simulink model "FOC_HF_G474"  (R2020b)
settings: Solver=FixedStepDiscrete  StartTime=0.0  StopTime=10  FixedStep=TsBSP  RelTol=1e-3
values from neighbouring files (symbols this model uses):
  BandwidthCurrentPI = 314.15926535897933    [G474_FOC_HF.sldd]
  Ld = 4.9E-5    [G474_FOC_HF.sldd]    (also in Hall_HFI_FOC_Data.sldd = 0.0004
  Ld_MODEL = 4.9E-5    [G474_FOC_HF.sldd]
  Lq = 4.9E-5    [G474_FOC_HF.sldd]    (also in Hall_HFI_FOC_Data.sldd = 0.00045
  Lq_MODEL = 4.9E-5    [G474_FOC_HF.sldd]
  MaxVoltage = 5.0    [G474_FOC_HF.sldd]
  PolePairs = 5.0    [G474_FOC_HF.sldd]
  PolePairs_MODEL = 5.0    [G474_FOC_HF.sldd]
  PWMHalfPeriod = 4199.0    [G474_FOC_HF.sldd]
  Rs = 0.082    [G474_FOC_HF.sldd]
  TsBSP = 2.0E-5    [G474_FOC_HF.sldd]
  TsFOC = 0.0001    [G474_FOC_HF.sldd]
  TsFOC_MODEL = 0.0001    [G474_FOC_HF.sldd]
undefined symbols (not defined in the file or in its folder): sigbuilder_block
libraries: pid_lib x4, mcbplantlib x1, autolibpmsminterior x1
(part 2 of 2)

== system FOC_HF_G474/FOC/FOC_CURRENT/SVPWM/CalcPWM/Switch Case Action Subsystem/tLimit ==
  t1 : Inport
  t2 : Inport  Port=2
  PWMHalfPeriod : Inport  Port=3
  If : If  IfExpression=u1
  If Action Subsystem : Subsystem  TreatAsAtomicUnit=on
  If Action Subsystem1 : Subsystem  TreatAsAtomicUnit=on
  Merge : Merge
  Merge1 : Merge
  Relational Operator : RelationalOperator  Operator=>  OutDataTypeStr=boolean  RndMeth=Simplest
  Sum4 : Sum  Inputs=|++
  t1Limit : Outport
  t2Limit : Outport  Port=2
  wires:
  t2/1 -> If Action Subsystem1/2(t2), If Action Subsystem/2(t2), Sum4/2
  Sum4/1 -> Relational Operator/1
  If/1 -> If Action Subsystem/Action
  Relational Operator/1 -> If/1
  PWMHalfPeriod/1 -> Relational Operator/2, If Action Subsystem/3(PWMHalfPeriod)
  t1/1 -> If Action Subsystem1/1(t1), If Action Subsystem/1(t1), Sum4/1
  If/2 -> If Action Subsystem1/Action
  If Action Subsystem/1(t1Limit) -> Merge/1
  If Action Subsystem1/1(t1Limit) -> Merge/2
  Merge/1 -> t1Limit/1
  If Action Subsystem1/2(t2Limit) -> Merge1/2
  If Action Subsystem/2(t2Limit) -> Merge1/1
  Merge1/1 -> t2Limit/1

== system FOC_HF_G474/FOC/FOC_CURRENT/SVPWM/CalcPWM/Switch Case Action Subsystem1/tLimit ==
  t2 : Inport
  t3 : Inport  Port=2
  PWMHalfPeriod : Inport  Port=3
  If : If  IfExpression=u1
  If Action Subsystem : Subsystem  TreatAsAtomicUnit=on
  If Action Subsystem1 : Subsystem  TreatAsAtomicUnit=on
  Merge : Merge
  Merge1 : Merge
  Relational Operator : RelationalOperator  Operator=>  OutDataTypeStr=boolean  RndMeth=Simplest
  Sum4 : Sum  Inputs=|++
  t2Limit : Outport
  t3Limit : Outport  Port=2
  wires:
  t3/1 -> If Action Subsystem1/2(t3), If Action Subsystem/2(t3), Sum4/2
  Sum4/1 -> Relational Operator/1
  If/1 -> If Action Subsystem/Action
  Relational Operator/1 -> If/1
  PWMHalfPeriod/1 -> Relational Operator/2, If Action Subsystem/3(PWMHalfPeriod)
  t2/1 -> If Action Subsystem1/1(t2), If Action Subsystem/1(t2), Sum4/1
  If/2 -> If Action Subsystem1/Action
  If Action Subsystem/1(t2Limit) -> Merge/1
  If Action Subsystem1/1(t2Limit) -> Merge/2
  Merge/1 -> t2Limit/1
  If Action Subsystem1/2(t3Limit) -> Merge1/2
  If Action Subsystem/2(t3Limit) -> Merge1/1
  Merge1/1 -> t3Limit/1

== system FOC_HF_G474/FOC/FOC_CURRENT/SVPWM/CalcPWM/Switch Case Action Subsystem2/tLimit ==
  t4 : Inport
  t3 : Inport  Port=2
  PWMHalfPeriod : Inport  Port=3
  If : If  IfExpression=u1
  If Action Subsystem : Subsystem  TreatAsAtomicUnit=on
  If Action Subsystem1 : Subsystem  TreatAsAtomicUnit=on
  Merge : Merge
  Merge1 : Merge
  Relational Operator : RelationalOperator  Operator=>  OutDataTypeStr=boolean  RndMeth=Simplest
  Sum4 : Sum  Inputs=|++
  t4Limit : Outport
  t3Limit : Outport  Port=2
  wires:
  t3/1 -> If Action Subsystem1/2(t3), If Action Subsystem/2(t3), Sum4/2
  Sum4/1 -> Relational Operator/1
  If/1 -> If Action Subsystem/Action
  Relational Operator/1 -> If/1
  PWMHalfPeriod/1 -> Relational Operator/2, If Action Subsystem/3(PWMHalfPeriod)
  t4/1 -> If Action Subsystem1/1(t4), If Action Subsystem/1(t4), Sum4/1
  If/2 -> If Action Subsystem1/Action
  If Action Subsystem/1(t4Limit) -> Merge/1
  If Action Subsystem1/1(t4Limit) -> Merge/2
  Merge/1 -> t4Limit/1
  If Action Subsystem1/2(t3Limit) -> Merge1/2
  If Action Subsystem/2(t3Limit) -> Merge1/1
  Merge1/1 -> t3Limit/1

== system FOC_HF_G474/FOC/FOC_CURRENT/SVPWM/CalcPWM/Switch Case Action Subsystem3/tLimit ==
  t4 : Inport
  t5 : Inport  Port=2
  PWMHalfPeriod : Inport  Port=3
  If : If  IfExpression=u1
  If Action Subsystem : Subsystem  TreatAsAtomicUnit=on
  If Action Subsystem1 : Subsystem  TreatAsAtomicUnit=on
  Merge : Merge
  Merge1 : Merge
  Relational Operator : RelationalOperator  Operator=>  OutDataTypeStr=boolean  RndMeth=Simplest
  Sum4 : Sum  Inputs=|++
  t4Limit : Outport
  t5Limit : Outport  Port=2
  wires:
  t5/1 -> If Action Subsystem1/2(t5), If Action Subsystem/2(t5), Sum4/2
  Sum4/1 -> Relational Operator/1
  If/1 -> If Action Subsystem/Action
  Relational Operator/1 -> If/1
  PWMHalfPeriod/1 -> Relational Operator/2, If Action Subsystem/3(PWMHalfPeriod)
  t4/1 -> If Action Subsystem1/1(t4), If Action Subsystem/1(t4), Sum4/1
  If/2 -> If Action Subsystem1/Action
  If Action Subsystem/1(t4Limit) -> Merge/1
  If Action Subsystem1/1(t4Limit) -> Merge/2
  Merge/1 -> t4Limit/1
  If Action Subsystem1/2(t5Limit) -> Merge1/2
  If Action Subsystem/2(t5Limit) -> Merge1/1
  Merge1/1 -> t5Limit/1

== system FOC_HF_G474/FOC/FOC_CURRENT/SVPWM/CalcPWM/Switch Case Action Subsystem4/tLimit ==
  t5 : Inport
  t6 : Inport  Port=2
  PWMHalfPeriod : Inport  Port=3
  If : If  IfExpression=u1
  If Action Subsystem : Subsystem  TreatAsAtomicUnit=on
  If Action Subsystem1 : Subsystem  TreatAsAtomicUnit=on
  Merge : Merge
  Merge1 : Merge
  Relational Operator : RelationalOperator  Operator=>  OutDataTypeStr=boolean  RndMeth=Simplest
  Sum4 : Sum  Inputs=|++
  t5Limit : Outport
  t6Limit : Outport  Port=2
  wires:
  t6/1 -> If Action Subsystem1/2(t6), If Action Subsystem/2(t6), Sum4/2
  Sum4/1 -> Relational Operator/1
  If/1 -> If Action Subsystem/Action
  Relational Operator/1 -> If/1
  PWMHalfPeriod/1 -> Relational Operator/2, If Action Subsystem/3(PWMHalfPeriod)
  t5/1 -> If Action Subsystem1/1(t5), If Action Subsystem/1(t5), Sum4/1
  If/2 -> If Action Subsystem1/Action
  If Action Subsystem/1(t5Limit) -> Merge/1
  If Action Subsystem1/1(t5Limit) -> Merge/2
  Merge/1 -> t5Limit/1
  If Action Subsystem1/2(t6Limit) -> Merge1/2
  If Action Subsystem/2(t6Limit) -> Merge1/1
  Merge1/1 -> t6Limit/1

== system FOC_HF_G474/FOC/FOC_CURRENT/SVPWM/CalcPWM/Switch Case Action Subsystem5/tLimit ==
  t1 : Inport
  t6 : Inport  Port=2
  PWMHalfPeriod : Inport  Port=3
  If : If  IfExpression=u1
  If Action Subsystem : Subsystem  TreatAsAtomicUnit=on
  If Action Subsystem1 : Subsystem  TreatAsAtomicUnit=on
  Merge : Merge
  Merge1 : Merge
  Relational Operator : RelationalOperator  Operator=>  OutDataTypeStr=boolean  RndMeth=Simplest
  Sum4 : Sum  Inputs=|++
  t1Limit : Outport
  t6Limit : Outport  Port=2
  wires:
  t6/1 -> If Action Subsystem1/2(t6), If Action Subsystem/2(t6), Sum4/2
  Sum4/1 -> Relational Operator/1
  If/1 -> If Action Subsystem/Action
  Relational Operator/1 -> If/1
  PWMHalfPeriod/1 -> Relational Operator/2, If Action Subsystem/3(PWMHalfPeriod)
  t1/1 -> If Action Subsystem1/1(t1), If Action Subsystem/1(t1), Sum4/1
  If/2 -> If Action Subsystem1/Action
  If Action Subsystem/1(t1Limit) -> Merge/1
  If Action Subsystem1/1(t1Limit) -> Merge/2
  Merge/1 -> t1Limit/1
  If Action Subsystem1/2(t6Limit) -> Merge1/2
  If Action Subsystem/2(t6Limit) -> Merge1/1
  Merge1/1 -> t6Limit/1

== system FOC_HF_G474/FOC/FOC_CURRENT/SVPWM/JudgeSector/If Action Subsystem/If Action Subsystem ==
  Valpha : Inport
  Vbeta : Inport  Port=2
  Action Port : ActionPort  ActionPortLabel=if(u1 )
  1/sqrt(3) : Gain  Gain=1/sqrt(3)
  Constant : Constant  Value=2  OutDataTypeStr=single  SampleTime=-1
  Constant1 : Constant  OutDataTypeStr=single
  Relational Operator : RelationalOperator  Operator=<  OutDataTypeStr=boolean  ZeroCross=off  RndMeth=Simplest
  Switch : Switch  Criteria=u2 > Threshold
  Sector : Outport
  wires:
  Vbeta/1 -> 1/sqrt(3)/1
  Relational Operator/1 -> Switch/2
  Valpha/1 -> Relational Operator/1
  1/sqrt(3)/1 -> Relational Operator/2
  Constant/1 -> Switch/1
  Constant1/1 -> Switch/3
  Switch/1 -> Sector/1

== system FOC_HF_G474/FOC/FOC_CURRENT/SVPWM/JudgeSector/If Action Subsystem/If Action Subsystem1 ==
  Valpha : Inport
  Vbeta : Inport  Port=2
  Action Port : ActionPort  ActionPortLabel=else
  -1/sqrt(3) : Gain  Gain=-1/sqrt(3)
  Constant : Constant  Value=3  OutDataTypeStr=single  SampleTime=-1
  Constant1 : Constant  Value=2  OutDataTypeStr=single  SampleTime=-1
  Relational Operator : RelationalOperator  Operator=<  OutDataTypeStr=boolean  RndMeth=Simplest
  Switch : Switch  Criteria=u2 > Threshold
  Sector : Outport
  wires:
  Vbeta/1 -> -1/sqrt(3)/1
  -1/sqrt(3)/1 -> Relational Operator/2
  Valpha/1 -> Relational Operator/1
  Relational Operator/1 -> Switch/2
  Switch/1 -> Sector/1
  Constant/1 -> Switch/1
  Constant1/1 -> Switch/3

== system FOC_HF_G474/FOC/FOC_CURRENT/SVPWM/JudgeSector/If Action Subsystem1/If Action Subsystem ==
  Valpha : Inport
  Vbeta : Inport  Port=2
  Action Port : ActionPort  ActionPortLabel=if(u1)
  -1/sqrt(3) : Gain  Gain=-1/sqrt(3)
  Constant : Constant  Value=5  OutDataTypeStr=single  SampleTime=-1
  Constant1 : Constant  Value=6  OutDataTypeStr=single
  Relational Operator : RelationalOperator  Operator=<  OutDataTypeStr=boolean  ZeroCross=off  RndMeth=Simplest
  Switch : Switch  Criteria=u2 > Threshold
  Sector : Outport
  wires:
  Vbeta/1 -> -1/sqrt(3)/1
  Relational Operator/1 -> Switch/2
  Valpha/1 -> Relational Operator/1
  -1/sqrt(3)/1 -> Relational Operator/2
  Constant/1 -> Switch/1
  Constant1/1 -> Switch/3
  Switch/1 -> Sector/1

== system FOC_HF_G474/FOC/FOC_CURRENT/SVPWM/JudgeSector/If Action Subsystem1/If Action Subsystem1 ==
  Valpha : Inport
  Vbeta : Inport  Port=2
  Action Port : ActionPort  ActionPortLabel=else
  1/sqrt(3) : Gain  Gain=1/sqrt(3)
  Constant : Constant  Value=4  OutDataTypeStr=single  SampleTime=-1
  Constant1 : Constant  Value=5  OutDataTypeStr=single  SampleTime=-1
  Relational Operator : RelationalOperator  Operator=<  OutDataTypeStr=boolean  RndMeth=Simplest
  Switch : Switch  Criteria=u2 > Threshold
  Sector : Outport
  wires:
  Vbeta/1 -> 1/sqrt(3)/1
  1/sqrt(3)/1 -> Relational Operator/2
  Valpha/1 -> Relational Operator/1
  Relational Operator/1 -> Switch/2
  Switch/1 -> Sector/1
  Constant/1 -> Switch/1
  Constant1/1 -> Switch/3

== system FOC_HF_G474/FOC/FOC_CURRENT/InjectSolve/PLL/SpeedToTheta/RangeLimit/If Action Subsystem ==
  In1 : Inport
  Action Port : ActionPort
  Constant : Constant  Value=2*pi  SampleTime=-1
  Sum : Sum  Inputs=|++
  Out1 : Outport
  wires:
  In1/1 -> Sum/1
  Constant/1 -> Sum/2
  Sum/1 -> Out1/1

== system FOC_HF_G474/FOC/FOC_CURRENT/InjectSolve/PLL/SpeedToTheta/RangeLimit/If Action Subsystem1 ==
  In1 : Inport
  Action Port : ActionPort
  Constant : Constant  Value=2*pi  SampleTime=-1
  Sum : Sum  Inputs=|+-
  Out1 : Outport
  wires:
  In1/1 -> Sum/1
  Constant/1 -> Sum/2
  Sum/1 -> Out1/1

== system FOC_HF_G474/FOC/FOC_CURRENT/InjectSolve/PLL/SpeedToTheta/RangeLimit/If Action Subsystem2 ==
  In1 : Inport
  Action Port : ActionPort
  Out1 : Outport
  wires:
  In1/1 -> Out1/1

== system FOC_HF_G474/FOC/FOC_CURRENT/InjectSolve/QPLL/SpeedToTheta/RangeLimit/If Action Subsystem ==
  In1 : Inport
  Action Port : ActionPort  ActionPortLabel=elseif(u2)
  Constant : Constant  Value=2*pi  OutDataTypeStr=single  SampleTime=-1
  Sum : Sum  Inputs=|++
  Out1 : Outport
  wires:
  In1/1 -> Sum/1
  Constant/1 -> Sum/2
  Sum/1 -> Out1/1

== system FOC_HF_G474/FOC/FOC_CURRENT/InjectSolve/QPLL/SpeedToTheta/RangeLimit/If Action Subsystem1 ==
  In1 : Inport
  Action Port : ActionPort  ActionPortLabel=if(u1)
  Constant : Constant  Value=2*pi  OutDataTypeStr=single  SampleTime=-1
  Sum : Sum  Inputs=|+-
  Out1 : Outport
  wires:
  In1/1 -> Sum/1
  Constant/1 -> Sum/2
  Sum/1 -> Out1/1

== system FOC_HF_G474/FOC/FOC_CURRENT/InjectSolve/QPLL/SpeedToTheta/RangeLimit/If Action Subsystem2 ==
  In1 : Inport
  Action Port : ActionPort  ActionPortLabel=else
  Out1 : Outport
  wires:
  In1/1 -> Out1/1

== system FOC_HF_G474/FOC/FOC_CURRENT/SVPWM/CalcPWM/Switch Case Action Subsystem/tLimit/If Action Subsystem ==
  t1 : Inport
  t2 : Inport  Port=2
  PWMHalfPeriod : Inport  Port=3
  Action Port : ActionPort  ActionPortLabel=if(u1)
  Divide : Product  Inputs=*/
  Product : Product
  Product1 : Product
  Sum : Sum  Inputs=|++
  t1Limit : Outport
  t2Limit : Outport  Port=2
  wires:
  t1/1 -> Product/2, Sum/1
  t2/1 -> Product1/2, Sum/2
  Sum/1 -> Divide/2
  PWMHalfPeriod/1 -> Divide/1
  Divide/1 -> Product1/1, Product/1
  Product/1 -> t1Limit/1
  Product1/1 -> t2Limit/1

== system FOC_HF_G474/FOC/FOC_CURRENT/SVPWM/CalcPWM/Switch Case Action Subsystem/tLimit/If Action Subsystem1 ==
  t1 : Inport
  t2 : Inport  Port=2
  Action Port : ActionPort  ActionPortLabel=else
  t1Limit : Outport
  t2Limit : Outport  Port=2
  wires:
  t1/1 -> t1Limit/1
  t2/1 -> t2Limit/1

== system FOC_HF_G474/FOC/FOC_CURRENT/SVPWM/CalcPWM/Switch Case Action Subsystem1/tLimit/If Action Subsystem ==
  t2 : Inport
  t3 : Inport  Port=2
  PWMHalfPeriod : Inport  Port=3
  Action Port : ActionPort  ActionPortLabel=if(u1)
  Divide : Product  Inputs=*/
  Product : Product
  Product1 : Product
  Sum : Sum  Inputs=|++
  t2Limit : Outport
  t3Limit : Outport  Port=2
  wires:
  t2/1 -> Product/2, Sum/1
  t3/1 -> Product1/2, Sum/2
  Sum/1 -> Divide/2
  PWMHalfPeriod/1 -> Divide/1
  Divide/1 -> Product1/1, Product/1
  Product/1 -> t2Limit/1
  Product1/1 -> t3Limit/1

== system FOC_HF_G474/FOC/FOC_CURRENT/SVPWM/CalcPWM/Switch Case Action Subsystem1/tLimit/If Action Subsystem1 ==
  t2 : Inport
  t3 : Inport  Port=2
  Action Port : ActionPort  ActionPortLabel=else
  t2Limit : Outport
  t3Limit : Outport  Port=2
  wires:
  t2/1 -> t2Limit/1
  t3/1 -> t3Limit/1

== system FOC_HF_G474/FOC/FOC_CURRENT/SVPWM/CalcPWM/Switch Case Action Subsystem2/tLimit/If Action Subsystem ==
  t4 : Inport
  t3 : Inport  Port=2
  PWMHalfPeriod : Inport  Port=3
  Action Port : ActionPort  ActionPortLabel=if(u1)
  Divide : Product  Inputs=*/
  Product : Product
  Product1 : Product
  Sum : Sum  Inputs=|++
  t4Limit : Outport
  t3Limit : Outport  Port=2
  wires:
  t4/1 -> Product/2, Sum/1
  t3/1 -> Product1/2, Sum/2
  Sum/1 -> Divide/2
  PWMHalfPeriod/1 -> Divide/1
  Divide/1 -> Product1/1, Product/1
  Product/1 -> t4Limit/1
  Product1/1 -> t3Limit/1

== system FOC_HF_G474/FOC/FOC_CURRENT/SVPWM/CalcPWM/Switch Case Action Subsystem2/tLimit/If Action Subsystem1 ==
  t4 : Inport
  t3 : Inport  Port=2
  Action Port : ActionPort  ActionPortLabel=else
  t4Limit : Outport
  t3Limit : Outport  Port=2
  wires:
  t4/1 -> t4Limit/1
  t3/1 -> t3Limit/1

== system FOC_HF_G474/FOC/FOC_CURRENT/SVPWM/CalcPWM/Switch Case Action Subsystem3/tLimit/If Action Subsystem ==
  t4 : Inport
  t5 : Inport  Port=2
  PWMHalfPeriod : Inport  Port=3
  Action Port : ActionPort  ActionPortLabel=if(u1)
  Divide : Product  Inputs=*/
  Product : Product
  Product1 : Product
  Sum : Sum  Inputs=|++
  t4Limit : Outport
  t5Limit : Outport  Port=2
  wires:
  t4/1 -> Product/2, Sum/1
  t5/1 -> Product1/2, Sum/2
  Sum/1 -> Divide/2
  PWMHalfPeriod/1 -> Divide/1
  Divide/1 -> Product1/1, Product/1
  Product/1 -> t4Limit/1
  Product1/1 -> t5Limit/1

== system FOC_HF_G474/FOC/FOC_CURRENT/SVPWM/CalcPWM/Switch Case Action Subsystem3/tLimit/If Action Subsystem1 ==
  t4 : Inport
  t5 : Inport  Port=2
  Action Port : ActionPort  ActionPortLabel=else
  t4Limit : Outport
  t5Limit : Outport  Port=2
  wires:
  t4/1 -> t4Limit/1
  t5/1 -> t5Limit/1

== system FOC_HF_G474/FOC/FOC_CURRENT/SVPWM/CalcPWM/Switch Case Action Subsystem4/tLimit/If Action Subsystem ==
  t5 : Inport
  t6 : Inport  Port=2
  PWMHalfPeriod : Inport  Port=3
  Action Port : ActionPort  ActionPortLabel=if(u1)
  Divide : Product  Inputs=*/
  Product : Product
  Product1 : Product
  Sum : Sum  Inputs=|++
  t5Limit : Outport
  t6Limit : Outport  Port=2
  wires:
  t5/1 -> Product/2, Sum/1
  t6/1 -> Product1/2, Sum/2
  Sum/1 -> Divide/2
  PWMHalfPeriod/1 -> Divide/1
  Divide/1 -> Product1/1, Product/1
  Product/1 -> t5Limit/1
  Product1/1 -> t6Limit/1

== system FOC_HF_G474/FOC/FOC_CURRENT/SVPWM/CalcPWM/Switch Case Action Subsystem4/tLimit/If Action Subsystem1 ==
  t5 : Inport
  t6 : Inport  Port=2
  Action Port : ActionPort  ActionPortLabel=else
  t5Limit : Outport
  t6Limit : Outport  Port=2
  wires:
  t5/1 -> t5Limit/1
  t6/1 -> t6Limit/1

== system FOC_HF_G474/FOC/FOC_CURRENT/SVPWM/CalcPWM/Switch Case Action Subsystem5/tLimit/If Action Subsystem ==
  t1 : Inport
  t6 : Inport  Port=2
  PWMHalfPeriod : Inport  Port=3
  Action Port : ActionPort  ActionPortLabel=if(u1)
  Divide : Product  Inputs=*/
  Product : Product
  Product1 : Product
  Sum : Sum  Inputs=|++
  t1Limit : Outport
  t6Limit : Outport  Port=2
  wires:
  t1/1 -> Product/2, Sum/1
  t6/1 -> Product1/2, Sum/2
  Sum/1 -> Divide/2
  PWMHalfPeriod/1 -> Divide/1
  Divide/1 -> Product1/1, Product/1
  Product/1 -> t1Limit/1
  Product1/1 -> t6Limit/1

== system FOC_HF_G474/FOC/FOC_CURRENT/SVPWM/CalcPWM/Switch Case Action Subsystem5/tLimit/If Action Subsystem1 ==
  t1 : Inport
  t6 : Inport  Port=2
  Action Port : ActionPort  ActionPortLabel=else
  t1Limit : Outport
  t6Limit : Outport  Port=2
  wires:
  t1/1 -> t1Limit/1
  t6/1 -> t6Limit/1
